simulink model "CF025A_GmFctDiArbn"  (R2013b)
settings: Solver=FixedStepDiscrete  SolverMode=SingleTasking  StartTime=0.0  StopTime=60  FixedStep=0.002  RelTol=1e-3
values from neighbouring files (symbols this model uses):
  GmFctDiArbnEotHwAgThd = DataDict.Calibration    [CF025A_GmFctDiArbn_DataDict.m]
  GmFctDiArbnEotTi = DataDict.Calibration    [CF025A_GmFctDiArbn_DataDict.m]
  GmFctDiArbnOnCentrHwAgThd = DataDict.Calibration    [CF025A_GmFctDiArbn_DataDict.m]
  GmFctDiArbnOnCentrHwTqThd = DataDict.Calibration    [CF025A_GmFctDiArbn_DataDict.m]
  GmFctDiArbnOnCentrTi = DataDict.Calibration    [CF025A_GmFctDiArbn_DataDict.m]
  GmFctDiArbnSrvTi = DataDict.Calibration    [CF025A_GmFctDiArbn_DataDict.m]
  MICROSECTOSEC_ULS_F32 = DataDict.Constant    [CF025A_GmFctDiArbn_DataDict.m]
  ZEROHWAG_HWDEG_F32 = DataDict.Constant    [CF025A_GmFctDiArbn_DataDict.m]
undefined symbols (not defined in the file or in its folder): GmFctDiArbnSts1, LoaSt1
libraries: simulink x7, FixdToFloat x4
(part 1 of 3)
settings Model: Creator=QZWC4R  LastModifiedBy=QZWC4R
settings SolverCC: AutoInsertRateTranBlk=on  InsertRTBMode=Always
settings DataIOCC: LimitDataPoints=off  SaveFormat=Structure  ReturnWorkspaceOutputs=on
settings OptimizationCC: BlockReduction=off  InlineParams=on  ZeroExternalMemoryAtStartup=off  ZeroInternalMemoryAtStartup=off  OptimizeModelRefInitCode=on  LifeSpan=1
settings DebuggingCC: SignalInfNanChecking=error  SignalRangeChecking=warning  UnderspecifiedInitializationDetection=Simplified  SolverPrmCheckMsg=error  InheritedTsInSrcMsg=error  DiscreteInheritContinuousMsg=error  SingleTaskRateTransMsg=error  TasksWithSamePriorityMsg=error  SigSpecEnsureSampleTimeMsg=error  CheckMatrixSingularityMsg=error  ParameterUnderflowMsg=error  ParameterPrecisionLossMsg=error  ParameterTunabilityLossMsg=error  FixptConstUnderflowMsg=warning  FixptConstOverflowMsg=warning  VectorMatrixConversionMsg=error  SignalLabelMismatchMsg=error  UnconnectedInputMsg=error  UnconnectedOutputMsg=error  UnconnectedLineMsg=error  SFcnCompatibilityMsg=error  UniqueDataStoreMsg=warning  BusObjectLabelMismatch=error  RootOutportRequireBusObject=error  AssertControl=DisableAll  ModelReferenceIOMsg=error  ModelReferenceVersionMismatchMessage=warning  ModelReferenceIOMismatchMessage=error  ModelReferenceCSMismatchMessage=warning  ModelReferenceDataLoggingMessage=error  StateNameClashWarn=warning  StrictBusMsg=ErrorOnBusTreatedAsVector  NonBusSignalsTreatedAsBus=error  SFUnexpectedBacktrackingDiag=error  SFInvalidInputDataAccessInChartInitDiag=error  SFNoUnconditionalDefaultTransitionDiag=error  SFTransitionOutsideNaturalParentDiag=error  SFUnconditionalTransitionShadowingDiag=error  SFUndirectedBroadcastEventsDiag=error
settings ModelReferenceCC: ModelReferenceNumInstancesAllowed=Single
settings RTWCC: SystemTargetFile=autosar.tlc  GenCodeOnly=on  TemplateMakefile=ert_default_tmf  Description=AUTOSAR  GenerateReport=on  ProcessScript=autosar_make_rtw_hook  LaunchReport=on
settings CodeAppCC: GenerateComments=off  IgnoreCustomStorageClasses=off  CustomSymbolStrType=$N$R$M  CustomSymbolStrBlkIO=$N$M  SimulinkBlockComments=off
settings STFCustomTargetCC: ParMdlRefBuildCompliant=on  CompOptLevelCompliant=on  IncludeMdlTerminateFcn=off  CombineOutputUpdateFcns=on  SuppressErrorStatus=on  ERTFirstTimeCompliant=on  ERTCustomFileBanners=on  SupportNonFinite=off  SupportComplex=off  SupportContinuousTime=off  SupportNonInlinedSFcns=off  MATLABClassNameForMDSCustomization=Simulink.SoftwareTarget.ERTCustomization  AutosarCompliant=on  GRTInterface=off  SystemTargetFile=autosar.tlc
settings ERTTargetCC: CodeReplacementLibrary=ANSI_C  ConcurrentExecutionCompliant=off  IncludeMdlTerminateFcn=off  SuppressErrorStatus=on  SupportNonFinite=off  SupportComplex=off  ModelStepFunctionPrototypeControlCompliant=off  CPPClassGenCompliant=off  AutosarCompliant=on  InlinedParameterPlacement=NonHierarchical  ERTCustomFileTemplate=example_file_process.tlc  EnableUserReplacementTypes=on

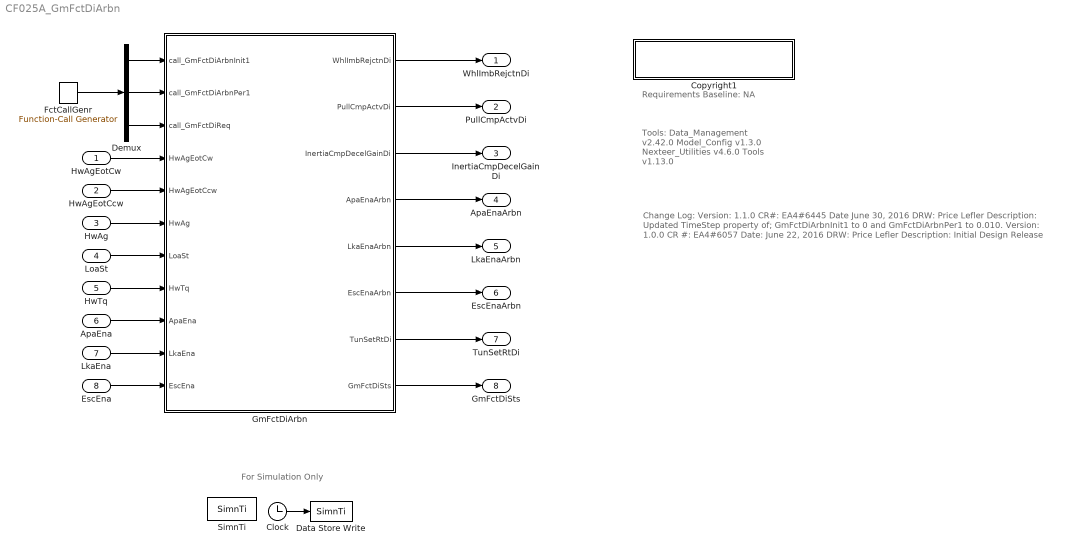
== system CF025A_GmFctDiArbn ==
  note: For Simulation Only
  note: Requirements Baseline:
      | NA
  note: Tools:
      | Data_Management v2.42.0
      | Model_Config v1.3.0
      | Nexteer_Utilities v4.6.0
      | Tools v1.13.0
  note: Change Log:
      |
      | Version: 1.1.0
      | CR#: EA4#6445
      | Date June 30, 2016
      | DRW: Price Lefler
      | Description:
      | 	Updated TimeStep property of; GmFctDiArbnInit1 to 0 and GmFctDiArbnPer1 to 0.010.
      |
      |
      | Version: 1.0.0
      | CR #: EA4#6057
      | Date: June 22, 2016
      | DRW: Price Lefler
      | Description:
      | 	Initial Design Release
  HwAgEotCw : Inport
  HwAgEotCcw : Inport  Port=2
  HwAg : Inport  Port=3
  LoaSt : Inport  Port=4
  HwTq : Inport  Port=5
  ApaEna : Inport  RequirementInfo={'linktype_rmi_doors' '0000bee1 (/E-STEER_New2/Subsytem Spec Documents/Subsystem Core Specs/Customer Functions CF FDR/CF-09 GM Overlay State Handler)' '#42' 'true' '2.1.0-3 GMOSH shall accept an input of an Automated Park Assist 2 Req' '' } %GIDa_2f26ec7d_8ce6_4a1b_a678_32b752ffef3f  Port=6
  LkaEna : Inport  RequirementInfo={'linktype_rmi_doors' '0000bee1 (/E-STEER_New2/Subsytem Spec Documents/Subsystem Core Specs/Customer Functions CF FDR/CF-09 GM Overlay State Handler)' '#48' 'true' '2.1.0-9 GMOSH shall accept an input of a Lane Keeping Assist Request ' '' } %GIDa_32a3aad7_3110_404c_9c6a_95ffa6fb6158  Port=7
  EscEna : Inport  RequirementInfo={'linktype_rmi_doors' '0000bee1 (/E-STEER_New2/Subsytem Spec Documents/Subsystem Core Specs/Customer Functions CF FDR/CF-09 GM Overlay State Handler)' '#51' 'true' '2.1.0-12 GMOSH shall accept an input for a Stability Control Enhanceme' '' } %GIDa_bf71266e_d5fd_41ad_bffd_97b37bc2a8a3  Port=8
  Clock : Clock
  Copyright1 : Subsystem  Description=|  mask(Copyright Information){none=on}
      | Copyright info block.                                               
      |                                                                     
      | Place copyright information at the top of every subsystem in design.
      mask prompts: none "No parameters"
      mask help: Place copyright information at the top of every subsystem in design.
      mask Display:
      | NxtrConf = 'Nexteer Confidential';
      | 
      | sys = bdroot; %handle for the current model ("system")
      | first = get_param(sys,'Created');
      | if(isempty(first))
      |     first = datestr(now,'yyyy');
      | else
      |     first = first(end-3:end);  %year is last four digits
      | end
      | 
      | last = get_param(sys,'LastModifiedDate');
      | if isempty(last)
      |     last = datestr(now,'yyyy');
      | else
      |     last = last(end-3:end);
      | end
      | 
      | if strcmp(first,last)
      |     fprintf('%s\nCopyright  %s Nexteer',NxtrConf,first);
      | else
      |     fprintf('%s\n%s%s-%s Nexteer',NxtrConf,char(169),first,last);
      | end
  Data Store Write : DataStoreWrite  DataStoreName=SimnTi
  Demux : Demux  Outputs=3
  FctCallGenr : simulink/Ports & Subsystems/Function-Call Generator  sample_time=0.010  numberOfIterations=1
  GmFctDiArbn : Subsystem
  SimnTi : DataStoreMemory  DataStoreName=SimnTi
  WhlImbRejctnDi : Outport
  PullCmpActvDi : Outport  Port=2
  InertiaCmpDecelGainDi : Outport  Port=3
  ApaEnaArbn : Outport  Port=4
  LkaEnaArbn : Outport  Port=5
  EscEnaArbn : Outport  Port=6
  TunSetRtDi : Outport  Port=7
  GmFctDiSts : Outport  Port=8
  wires:
  Clock/1 -> Data Store Write/1
  GmFctDiArbn/1(WhlImbRejctnDi) -> WhlImbRejctnDi/1
  GmFctDiArbn/2(PullCmpActvDi) -> PullCmpActvDi/1
  GmFctDiArbn/4(ApaEnaArbn) -> ApaEnaArbn/1
  GmFctDiArbn/5(LkaEnaArbn) -> LkaEnaArbn/1
  GmFctDiArbn/6(EscEnaArbn) -> EscEnaArbn/1
  GmFctDiArbn/7(TunSetRtDi) -> TunSetRtDi/1
  GmFctDiArbn/8(GmFctDiSts) -> GmFctDiSts/1
  HwAgEotCw/1 -> GmFctDiArbn/4(HwAgEotCw)
  HwAgEotCcw/1 -> GmFctDiArbn/5(HwAgEotCcw)
  HwAg/1 -> GmFctDiArbn/6(HwAg)
  LoaSt/1 -> GmFctDiArbn/7(LoaSt)
  HwTq/1 -> GmFctDiArbn/8(HwTq)
  ApaEna/1 -> GmFctDiArbn/9(ApaEna)
  LkaEna/1 -> GmFctDiArbn/10(LkaEna)
  EscEna/1 -> GmFctDiArbn/11(EscEna)
  GmFctDiArbn/3(InertiaCmpDecelGainDi) -> InertiaCmpDecelGainDi/1
  Demux/1 -> GmFctDiArbn/1(call_GmFctDiArbnInit1)
  Demux/2 -> GmFctDiArbn/2(call_GmFctDiArbnPer1)
  Demux/3 -> GmFctDiArbn/3(call_GmFctDiReq)
  FctCallGenr/1 -> Demux/1

== system CF025A_GmFctDiArbn/Copyright1 ==

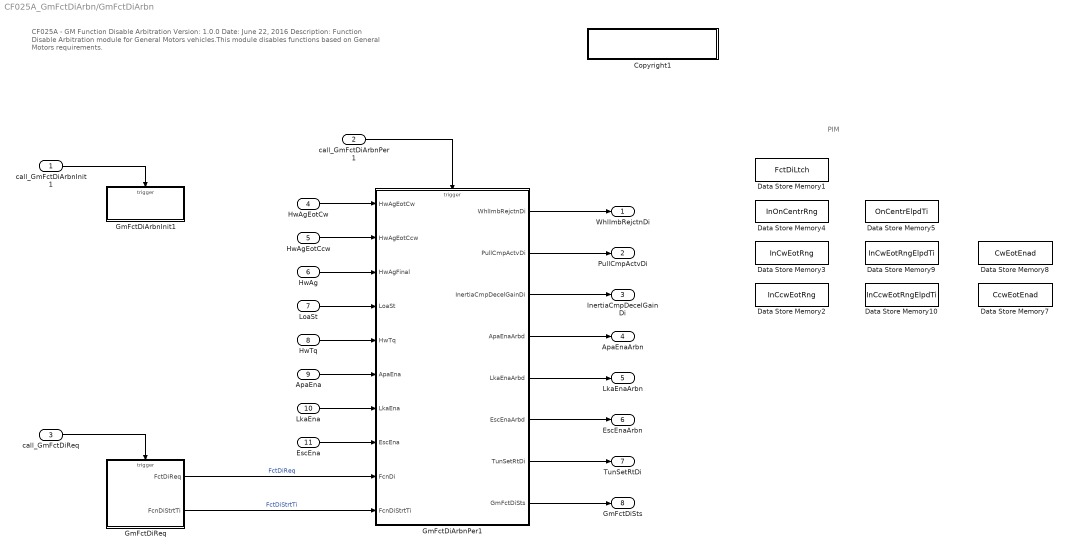
== system CF025A_GmFctDiArbn/GmFctDiArbn ==
  note: CF025A - GM Function Disable Arbitration
      | Version: 1.0.0
      | Date: June 22, 2016
      | Description:
      | 	 Function Disable Arbitration module for General Motors vehicles.This module disables functions based on General Motors requirements.
  note: PIM
  call_GmFctDiArbnInit1 : Inport
  call_GmFctDiArbnPer1 : Inport  Port=2
  call_GmFctDiReq : Inport  Port=3
  HwAgEotCw : Inport  Port=4
  HwAgEotCcw : Inport  Port=5
  HwAg : Inport  Port=6
  LoaSt : Inport  Port=7
  HwTq : Inport  Port=8
  ApaEna : Inport  RequirementInfo={'linktype_rmi_doors' '0000bee1 (/E-STEER_New2/Subsytem Spec Documents/Subsystem Core Specs/Customer Functions CF FDR/CF-09 GM Overlay State Handler)' '#42' 'true' '2.1.0-3 GMOSH shall accept an input of an Automated Park Assist 2 Req' '' } %GIDa_2c17c048_e723_4115_94ae_0e322b12958e  Port=9
  LkaEna : Inport  RequirementInfo={'linktype_rmi_doors' '0000bee1 (/E-STEER_New2/Subsytem Spec Documents/Subsystem Core Specs/Customer Functions CF FDR/CF-09 GM Overlay State Handler)' '#48' 'true' '2.1.0-9 GMOSH shall accept an input of a Lane Keeping Assist Request ' '' } %GIDa_a26b014d_6879_4602_9502_03f06376d044  Port=10
  EscEna : Inport  RequirementInfo={'linktype_rmi_doors' '0000bee1 (/E-STEER_New2/Subsytem Spec Documents/Subsystem Core Specs/Customer Functions CF FDR/CF-09 GM Overlay State Handler)' '#51' 'true' '2.1.0-12 GMOSH shall accept an input for a Stability Control Enhanceme' '' } %GIDa_8379b319_8fa0_4ff7_8623_9b680c80b153  Port=11
  Copyright1 : Subsystem  Description=|  mask(Copyright Information){none=on}
      | Copyright info block.                                               
      |                                                                     
      | Place copyright information at the top of every subsystem in design.
      mask prompts: none "No parameters"
      mask help: Place copyright information at the top of every subsystem in design.
      mask Display:
      | NxtrConf = 'Nexteer Confidential';
      | 
      | sys = bdroot; %handle for the current model ("system")
      | first = get_param(sys,'Created');
      | if(isempty(first))
      |     first = datestr(now,'yyyy');
      | else
      |     first = first(end-3:end);  %year is last four digits
      | end
      | 
      | last = get_param(sys,'LastModifiedDate');
      | if isempty(last)
      |     last = datestr(now,'yyyy');
      | else
      |     last = last(end-3:end);
      | end
      | 
      | if strcmp(first,last)
      |     fprintf('%s\nCopyright  %s Nexteer',NxtrConf,first);
      | else
      |     fprintf('%s\n%s%s-%s Nexteer',NxtrConf,char(169),first,last);
      | end
  Data Store Memory1 : DataStoreMemory  DataStoreName=FctDiLtch  StateMustResolveToSignalObject=on
  Data Store Memory10 : DataStoreMemory  DataStoreName=InCcwEotRngElpdTi  StateMustResolveToSignalObject=on
  Data Store Memory2 : DataStoreMemory  DataStoreName=InCcwEotRng  StateMustResolveToSignalObject=on
  Data Store Memory3 : DataStoreMemory  DataStoreName=InCwEotRng  StateMustResolveToSignalObject=on
  Data Store Memory4 : DataStoreMemory  DataStoreName=InOnCentrRng  StateMustResolveToSignalObject=on
  Data Store Memory5 : DataStoreMemory  DataStoreName=OnCentrElpdTi  StateMustResolveToSignalObject=on
  Data Store Memory7 : DataStoreMemory  DataStoreName=CcwEotEnad  StateMustResolveToSignalObject=on
  Data Store Memory8 : DataStoreMemory  DataStoreName=CwEotEnad  StateMustResolveToSignalObject=on
  Data Store Memory9 : DataStoreMemory  DataStoreName=InCwEotRngElpdTi  StateMustResolveToSignalObject=on
  GmFctDiArbnInit1 : Subsystem  TreatAsAtomicUnit=on
  GmFctDiArbnPer1 : Subsystem  TreatAsAtomicUnit=on
  GmFctDiReq : Subsystem  TreatAsAtomicUnit=on
  WhlImbRejctnDi : Outport
  PullCmpActvDi : Outport  Port=2
  InertiaCmpDecelGainDi : Outport  Port=3
  ApaEnaArbn : Outport  Port=4
  LkaEnaArbn : Outport  Port=5
  EscEnaArbn : Outport  Port=6
  TunSetRtDi : Outport  Port=7
  GmFctDiSts : Outport  Port=8
  wires:
  call_GmFctDiArbnInit1/1 -> GmFctDiArbnInit1/Trigger
  call_GmFctDiArbnPer1/1 -> GmFctDiArbnPer1/Trigger
  HwTq/1 -> GmFctDiArbnPer1/5(HwTq)
  LoaSt/1 -> GmFctDiArbnPer1/4(LoaSt)
  HwAg/1 -> GmFctDiArbnPer1/3(HwAgFinal)
  HwAgEotCcw/1 -> GmFctDiArbnPer1/2(HwAgEotCcw)
  HwAgEotCw/1 -> GmFctDiArbnPer1/1(HwAgEotCw)
  GmFctDiArbnPer1/1(WhlImbRejctnDi) -> WhlImbRejctnDi/1
  GmFctDiArbnPer1/2(PullCmpActvDi) -> PullCmpActvDi/1
  GmFctDiArbnPer1/3(InertiaCmpDecelGainDi) -> InertiaCmpDecelGainDi/1
  GmFctDiArbnPer1/4(ApaEnaArbd) -> ApaEnaArbn/1
  GmFctDiArbnPer1/5(LkaEnaArbd) -> LkaEnaArbn/1
  GmFctDiArbnPer1/6(EscEnaArbd) -> EscEnaArbn/1
  call_GmFctDiReq/1 -> GmFctDiReq/Trigger
  GmFctDiReq/1(FctDiReq) -> GmFctDiArbnPer1/9(FcnDi)  "FctDiReq"
  ApaEna/1 -> GmFctDiArbnPer1/6(ApaEna)
  LkaEna/1 -> GmFctDiArbnPer1/7(LkaEna)
  EscEna/1 -> GmFctDiArbnPer1/8(EscEna)
  GmFctDiArbnPer1/7(TunSetRtDi) -> TunSetRtDi/1
  GmFctDiArbnPer1/8(GmFctDiSts) -> GmFctDiSts/1
  GmFctDiReq/2(FcnDiStrtTi) -> GmFctDiArbnPer1/10(FcnDiStrtTi)  "FctDiStrtTi"

== system CF025A_GmFctDiArbn/GmFctDiArbn/Copyright1 ==

== system CF025A_GmFctDiArbn/GmFctDiArbn/GmFctDiArbnInit1 ==
  function : TriggerPort  TriggerType=function-call
  Copyright1 : Subsystem  Description=|  mask(Copyright Information){none=on}
      | Copyright info block.                                               
      |                                                                     
      | Place copyright information at the top of every subsystem in design.
      mask prompts: none "No parameters"
      mask help: Place copyright information at the top of every subsystem in design.
      mask Display:
      | NxtrConf = 'Nexteer Confidential';
      | 
      | sys = bdroot; %handle for the current model ("system")
      | first = get_param(sys,'Created');
      | if(isempty(first))
      |     first = datestr(now,'yyyy');
      | else
      |     first = first(end-3:end);  %year is last four digits
      | end
      | 
      | last = get_param(sys,'LastModifiedDate');
      | if isempty(last)
      |     last = datestr(now,'yyyy');
      | else
      |     last = last(end-3:end);
      | end
      | 
      | if strcmp(first,last)
      |     fprintf('%s\nCopyright  %s Nexteer',NxtrConf,first);
      | else
      |     fprintf('%s\n%s%s-%s Nexteer',NxtrConf,char(169),first,last);
      | end

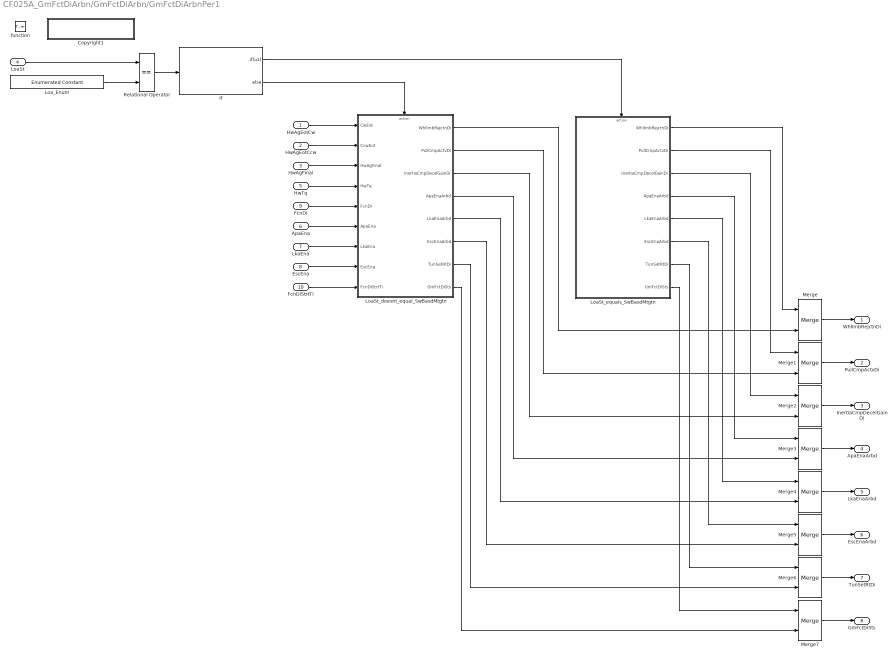
== system CF025A_GmFctDiArbn/GmFctDiArbn/GmFctDiArbnPer1 ==
  HwAgEotCw : Inport
  HwAgEotCcw : Inport  Port=2
  HwAgFinal : Inport  Port=3
  LoaSt : Inport  Port=4
  HwTq : Inport  Port=5
  ApaEna : Inport  RequirementInfo={'linktype_rmi_doors' '0000bee1 (/E-STEER_New2/Subsytem Spec Documents/Subsystem Core Specs/Customer Functions CF FDR/CF-09 GM Overlay State Handler)' '#42' 'true' '2.1.0-3 GMOSH shall accept an input of an Automated Park Assist 2 Req' '' } %GIDa_eb388981_6ca0_4296_8e81_aef3a122a5ab  Port=6
  LkaEna : Inport  RequirementInfo={'linktype_rmi_doors' '0000bee1 (/E-STEER_New2/Subsytem Spec Documents/Subsystem Core Specs/Customer Functions CF FDR/CF-09 GM Overlay State Handler)' '#48' 'true' '2.1.0-9 GMOSH shall accept an input of a Lane Keeping Assist Request ' '' } %GIDa_cd443268_1945_4186_bec6_c8c383fdf52f  Port=7
  EscEna : Inport  RequirementInfo={'linktype_rmi_doors' '0000bee1 (/E-STEER_New2/Subsytem Spec Documents/Subsystem Core Specs/Customer Functions CF FDR/CF-09 GM Overlay State Handler)' '#51' 'true' '2.1.0-12 GMOSH shall accept an input for a Stability Control Enhanceme' '' } %GIDa_e4a9320c_e488_484d_a205_861b0d5f4219  Port=8
  FcnDi : Inport  Port=9
  FcnDiStrtTi : Inport  Port=10  OutDataTypeStr=uint32
  function : TriggerPort  TriggerType=function-call
  Copyright1 : Subsystem  Description=|  mask(Copyright Information){none=on}
      | Copyright info block.                                               
      |                                                                     
      | Place copyright information at the top of every subsystem in design.
      mask prompts: none "No parameters"
      mask help: Place copyright information at the top of every subsystem in design.
      mask Display:
      | NxtrConf = 'Nexteer Confidential';
      | 
      | sys = bdroot; %handle for the current model ("system")
      | first = get_param(sys,'Created');
      | if(isempty(first))
      |     first = datestr(now,'yyyy');
      | else
      |     first = first(end-3:end);  %year is last four digits
      | end
      | 
      | last = get_param(sys,'LastModifiedDate');
      | if isempty(last)
      |     last = datestr(now,'yyyy');
      | else
      |     last = last(end-3:end);
      | end
      | 
      | if strcmp(first,last)
      |     fprintf('%s\nCopyright  %s Nexteer',NxtrConf,first);
      | else
      |     fprintf('%s\n%s%s-%s Nexteer',NxtrConf,char(169),first,last);
      | end
  If : If  IfExpression=u1
  LoaSt_doesnt_equal_SwBasdMtgtn : Subsystem  TreatAsAtomicUnit=on
  LoaSt_equals_SwBasdMtgtn : Subsystem  TreatAsAtomicUnit=on
  Loa_Enum : simulink/Sources/Enumerated Constant  OutDataTypeStr=Enum: LoaSt1  Value=LoaSt1.LOAST_SWBASDMTGTN  SampleTime=inf
  Merge{,1..7} (8 alike) : Merge
  Relational Operator : RelationalOperator  Operator===  OutDataTypeStr=boolean
  WhlImbRejctnDi : Outport
  PullCmpActvDi : Outport  Port=2
  InertiaCmpDecelGainDi : Outport  Port=3
  ApaEnaArbd : Outport  Port=4
  LkaEnaArbd : Outport  Port=5
  EscEnaArbd : Outport  Port=6
  TunSetRtDi : Outport  Port=7
  GmFctDiSts : Outport  Port=8
  wires:
  LoaSt/1 -> Relational Operator/1
  Loa_Enum/1 -> Relational Operator/2
  If/1 -> LoaSt_equals_SwBasdMtgtn/Action
  Merge/1 -> WhlImbRejctnDi/1
  Merge1/1 -> PullCmpActvDi/1
  Merge2/1 -> InertiaCmpDecelGainDi/1
  Merge3/1 -> ApaEnaArbd/1
  Merge4/1 -> LkaEnaArbd/1
  Merge5/1 -> EscEnaArbd/1
  If/2 -> LoaSt_doesnt_equal_SwBasdMtgtn/Action
  HwAgEotCw/1 -> LoaSt_doesnt_equal_SwBasdMtgtn/1(CwEot)
  HwAgEotCcw/1 -> LoaSt_doesnt_equal_SwBasdMtgtn/2(CcwEot)
  HwAgFinal/1 -> LoaSt_doesnt_equal_SwBasdMtgtn/3(HwAgFinal)
  HwTq/1 -> LoaSt_doesnt_equal_SwBasdMtgtn/4(HwTq)
  FcnDi/1 -> LoaSt_doesnt_equal_SwBasdMtgtn/5(FcnDi)
  ApaEna/1 -> LoaSt_doesnt_equal_SwBasdMtgtn/6(ApaEna)
  LkaEna/1 -> LoaSt_doesnt_equal_SwBasdMtgtn/7(LkaEna)
  EscEna/1 -> LoaSt_doesnt_equal_SwBasdMtgtn/8(EscEna)
  Merge6/1 -> TunSetRtDi/1
  Merge7/1 -> GmFctDiSts/1
  Relational Operator/1 -> If/1
  LoaSt_equals_SwBasdMtgtn/1(WhlImbRejctnDi) -> Merge/1
  LoaSt_doesnt_equal_SwBasdMtgtn/1(WhlImbRejctnDi) -> Merge/2
  LoaSt_equals_SwBasdMtgtn/2(PullCmpActvDi) -> Merge1/1
  LoaSt_doesnt_equal_SwBasdMtgtn/2(PullCmpActvDi) -> Merge1/2
  LoaSt_equals_SwBasdMtgtn/3(InertiaCmpDecelGainDi) -> Merge2/1
  LoaSt_doesnt_equal_SwBasdMtgtn/3(InertiaCmpDecelGainDi) -> Merge2/2
  LoaSt_equals_SwBasdMtgtn/4(ApaEnaArbd) -> Merge3/1
  LoaSt_doesnt_equal_SwBasdMtgtn/4(ApaEnaArbd) -> Merge3/2
  LoaSt_equals_SwBasdMtgtn/5(LkaEnaArbd) -> Merge4/1
  LoaSt_doesnt_equal_SwBasdMtgtn/5(LkaEnaArbd) -> Merge4/2
  LoaSt_equals_SwBasdMtgtn/6(EscEnaArbd) -> Merge5/1
  LoaSt_equals_SwBasdMtgtn/7(TunSetRtDi) -> Merge6/1
  LoaSt_doesnt_equal_SwBasdMtgtn/7(TunSetRtDi) -> Merge6/2
  LoaSt_doesnt_equal_SwBasdMtgtn/6(EscEnaArbd) -> Merge5/2
  LoaSt_equals_SwBasdMtgtn/8(GmFctDiSts) -> Merge7/1
  LoaSt_doesnt_equal_SwBasdMtgtn/8(GmFctDiSts) -> Merge7/2
  FcnDiStrtTi/1 -> LoaSt_doesnt_equal_SwBasdMtgtn/9(FcnDiStrtTi)

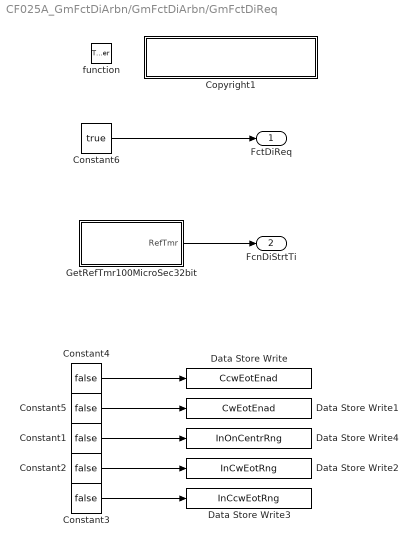
== system CF025A_GmFctDiArbn/GmFctDiArbn/GmFctDiReq ==
  function : TriggerPort  TriggerType=function-call
  Constant{1..5} (5 alike) : Constant  Value=false
  Constant6 : Constant  Value=true
  Copyright1 : Subsystem  Description=|  mask(Copyright Information){none=on}
      | Copyright info block.                                               
      |                                                                     
      | Place copyright information at the top of every subsystem in design.
      mask prompts: none "No parameters"
      mask help: Place copyright information at the top of every subsystem in design.
      mask Display:
      | NxtrConf = 'Nexteer Confidential';
      | 
      | sys = bdroot; %handle for the current model ("system")
      | first = get_param(sys,'Created');
      | if(isempty(first))
      |     first = datestr(now,'yyyy');
      | else
      |     first = first(end-3:end);  %year is last four digits
      | end
      | 
      | last = get_param(sys,'LastModifiedDate');
      | if isempty(last)
      |     last = datestr(now,'yyyy');
      | else
      |     last = last(end-3:end);
      | end
      | 
      | if strcmp(first,last)
      |     fprintf('%s\nCopyright  %s Nexteer',NxtrConf,first);
      | else
      |     fprintf('%s\n%s%s-%s Nexteer',NxtrConf,char(169),first,last);
      | end
  Data Store Write : DataStoreWrite  DataStoreName=CcwEotEnad
  Data Store Write1 : DataStoreWrite  DataStoreName=CwEotEnad
  Data Store Write2 : DataStoreWrite  DataStoreName=InCwEotRng
  Data Store Write3 : DataStoreWrite  DataStoreName=InCcwEotRng
  Data Store Write4 : DataStoreWrite  DataStoreName=InOnCentrRng
  GetRefTmr100MicroSec32bit : Subsystem
  FctDiReq : Outport  InitialOutput=false
      settings: AttributesFormatString=|
      | Output IC: %<InitialOutput>
      | For Simulation Only.
  FcnDiStrtTi : Outport  Port=2
  wires:
  GetRefTmr100MicroSec32bit/1(RefTmr) -> FcnDiStrtTi/1
  Constant4/1 -> Data Store Write/1
  Constant5/1 -> Data Store Write1/1
  Constant1/1 -> Data Store Write4/1
  Constant2/1 -> Data Store Write2/1
  Constant3/1 -> Data Store Write3/1
  Constant6/1 -> FctDiReq/1

== system CF025A_GmFctDiArbn/GmFctDiArbn/GmFctDiArbnInit1/Copyright1 ==

== system CF025A_GmFctDiArbn/GmFctDiArbn/GmFctDiArbnPer1/Copyright1 ==

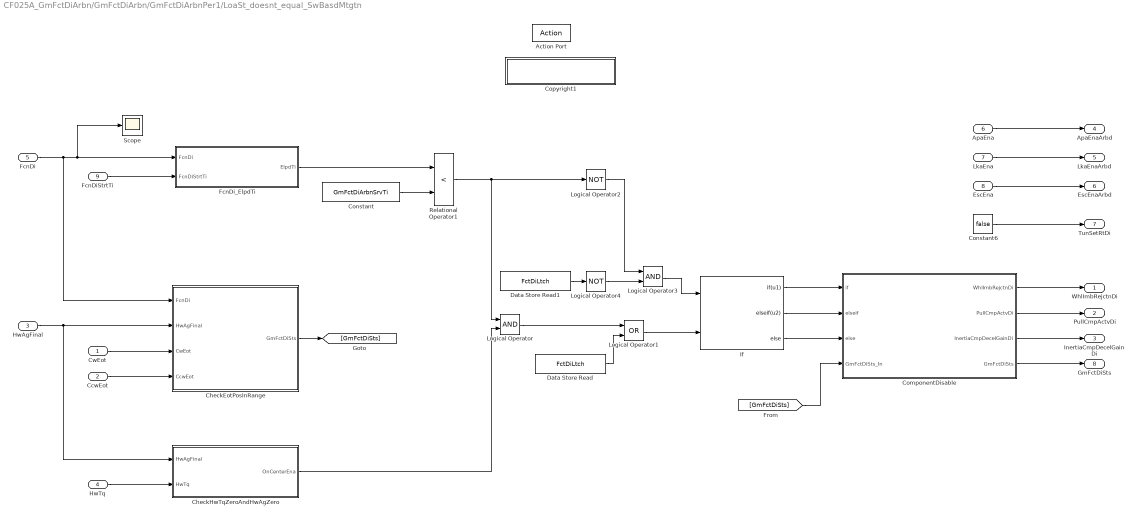
== system CF025A_GmFctDiArbn/GmFctDiArbn/GmFctDiArbnPer1/LoaSt_doesnt_equal_SwBasdMtgtn ==
  CwEot : Inport
  CcwEot : Inport  Port=2
  HwAgFinal : Inport  Port=3
  HwTq : Inport  Port=4
  FcnDi : Inport  Port=5
  ApaEna : Inport  RequirementInfo={'linktype_rmi_doors' '0000bee1 (/E-STEER_New2/Subsytem Spec Documents/Subsystem Core Specs/Customer Functions CF FDR/CF-09 GM Overlay State Handler)' '#42' 'true' '2.1.0-3 GMOSH shall accept an input of an Automated Park Assist 2 Req' '' } %GIDa_4c3b4a4d_4bd1_4ac6_b43d_6a3658ff9675  Port=6
  LkaEna : Inport  RequirementInfo={'linktype_rmi_doors' '0000bee1 (/E-STEER_New2/Subsytem Spec Documents/Subsystem Core Specs/Customer Functions CF FDR/CF-09 GM Overlay State Handler)' '#48' 'true' '2.1.0-9 GMOSH shall accept an input of a Lane Keeping Assist Request ' '' } %GIDa_aabf4122_7ea8_4387_9a0b_41aa0f5fdb39  Port=7
  EscEna : Inport  RequirementInfo={'linktype_rmi_doors' '0000bee1 (/E-STEER_New2/Subsytem Spec Documents/Subsystem Core Specs/Customer Functions CF FDR/CF-09 GM Overlay State Handler)' '#51' 'true' '2.1.0-12 GMOSH shall accept an input for a Stability Control Enhanceme' '' } %GIDa_db93f32a_9bac_4ded_8002_6031963bead0  Port=8
  FcnDiStrtTi : Inport  Port=9  OutDataTypeStr=uint32
  Action Port : ActionPort  ActionType=else
  CheckEotPosInRange : Subsystem
  CheckHwTqZeroAndHwAgZero : Subsystem
  ComponentDisable : Subsystem
  Constant : Constant  Value=GmFctDiArbnSrvTi
  Constant6 : Constant  Value=false  OutDataTypeStr=boolean
  Copyright1 : Subsystem  Description=|  mask(Copyright Information){none=on}
      | Copyright info block.                                               
      |                                                                     
      | Place copyright information at the top of every subsystem in design.
      mask prompts: none "No parameters"
      mask help: Place copyright information at the top of every subsystem in design.
      mask Display:
      | NxtrConf = 'Nexteer Confidential';
      | 
      | sys = bdroot; %handle for the current model ("system")
      | first = get_param(sys,'Created');
      | if(isempty(first))
      |     first = datestr(now,'yyyy');
      | else
      |     first = first(end-3:end);  %year is last four digits
      | end
      | 
      | last = get_param(sys,'LastModifiedDate');
      | if isempty(last)
      |     last = datestr(now,'yyyy');
      | else
      |     last = last(end-3:end);
      | end
      | 
      | if strcmp(first,last)
      |     fprintf('%s\nCopyright  %s Nexteer',NxtrConf,first);
      | else
      |     fprintf('%s\n%s%s-%s Nexteer',NxtrConf,char(169),first,last);
      | end
  Data Store Read : DataStoreRead  DataStoreName=FctDiLtch
  Data Store Read1 : DataStoreRead  DataStoreName=FctDiLtch
  FcnDi_ElpdTi : Subsystem
  If : If  NumInputs=2  IfExpression=u1  ElseIfExpressions=u2
  Logical Operator : Logic  AllPortsSameDT=off  OutDataTypeStr=boolean
  Logical Operator1 : Logic  Operator=OR  AllPortsSameDT=off  OutDataTypeStr=boolean
  Logical Operator2 : Logic  Operator=NOT  AllPortsSameDT=off  OutDataTypeStr=boolean
  Logical Operator3 : Logic  AllPortsSameDT=off  OutDataTypeStr=boolean
  Logical Operator4 : Logic  Operator=NOT  AllPortsSameDT=off  OutDataTypeStr=boolean
  Relational Operator1 : RelationalOperator  Operator=<  OutDataTypeStr=boolean
  Scope : Scope
      settings: SaveName=ScopeData5
  WhlImbRejctnDi : Outport
  PullCmpActvDi : Outport  Port=2
  InertiaCmpDecelGainDi : Outport  Port=3
  ApaEnaArbd : Outport  Port=4
  LkaEnaArbd : Outport  Port=5
  EscEnaArbd : Outport  Port=6
  TunSetRtDi : Outport  Port=7
  GmFctDiSts : Outport  Port=8
  wires:
  FcnDi_ElpdTi/1(ElpdTi) -> Relational Operator1/1
  CwEot/1 -> CheckEotPosInRange/3(CwEot)
  CcwEot/1 -> CheckEotPosInRange/4(CcwEot)
  HwAgFinal/1 -> CheckHwTqZeroAndHwAgZero/1(HwAgFinal), CheckEotPosInRange/2(HwAgFinal)
  HwTq/1 -> CheckHwTqZeroAndHwAgZero/2(HwTq)
  CheckHwTqZeroAndHwAgZero/1(OnCenterEna) -> Logical Operator/2
  Constant/1 -> Relational Operator1/2
  Relational Operator1/1 -> Logical Operator2/1, Logical Operator/1
  Logical Operator/1 -> Logical Operator1/1
  Logical Operator1/1 -> If/2
  Data Store Read/1 -> Logical Operator1/2
  ApaEna/1 -> ApaEnaArbd/1
  LkaEna/1 -> LkaEnaArbd/1
  EscEna/1 -> EscEnaArbd/1
  Constant6/1 -> TunSetRtDi/1
  If/1 -> ComponentDisable/1(if)
  If/2 -> ComponentDisable/2(elseif)
  If/3 -> ComponentDisable/3(else)
  ComponentDisable/1(WhlImbRejctnDi) -> WhlImbRejctnDi/1
  ComponentDisable/2(PullCmpActvDi) -> PullCmpActvDi/1
  ComponentDisable/3(InertiaCmpDecelGainDi) -> InertiaCmpDecelGainDi/1
  ComponentDisable/4(GmFctDiSts) -> GmFctDiSts/1
  CheckEotPosInRange/1(GmFctDiSts) -> [GmFctDiSts]
  [GmFctDiSts] -> ComponentDisable/4(GmFctDiSts_In)
  FcnDiStrtTi/1 -> FcnDi_ElpdTi/2(FcnDiStrtTi)
  Data Store Read1/1 -> Logical Operator4/1
  Logical Operator4/1 -> Logical Operator3/2
  FcnDi/1 -> Scope/1, FcnDi_ElpdTi/1(FcnDi), CheckEotPosInRange/1(FcnDi)
  Logical Operator2/1 -> Logical Operator3/1
  Logical Operator3/1 -> If/1

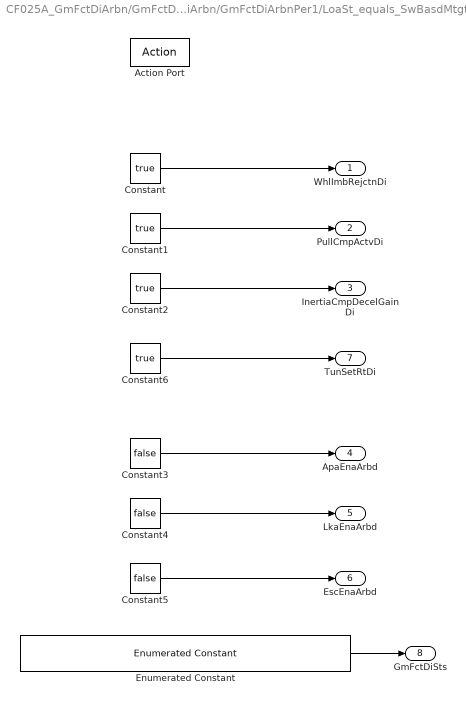
== system CF025A_GmFctDiArbn/GmFctDiArbn/GmFctDiArbnPer1/LoaSt_equals_SwBasdMtgtn ==
  Action Port : ActionPort  ActionType=then
  Constant{,1..2,6} (4 alike) : Constant  Value=true  OutDataTypeStr=boolean
  Constant3 : Constant  Value=false  OutDataTypeStr=boolean
  Constant4 : Constant  Value=false  OutDataTypeStr=boolean
  Constant5 : Constant  Value=false  OutDataTypeStr=boolean
  Enumerated Constant : simulink/Sources/Enumerated Constant  OutDataTypeStr=Enum: GmFctDiArbnSts1  Value=GmFctDiArbnSts1.GMFCTDIARBNSTS_SWBASDMTGTNFAIL  SampleTime=inf
  WhlImbRejctnDi : Outport
  PullCmpActvDi : Outport  Port=2
  InertiaCmpDecelGainDi : Outport  Port=3
  ApaEnaArbd : Outport  Port=4
  LkaEnaArbd : Outport  Port=5
  EscEnaArbd : Outport  Port=6
  TunSetRtDi : Outport  Port=7
  GmFctDiSts : Outport  Port=8
  wires:
  Constant/1 -> WhlImbRejctnDi/1
  Constant1/1 -> PullCmpActvDi/1
  Constant2/1 -> InertiaCmpDecelGainDi/1
  Constant3/1 -> ApaEnaArbd/1
  Constant4/1 -> LkaEnaArbd/1
  Constant5/1 -> EscEnaArbd/1
  Constant6/1 -> TunSetRtDi/1
  Enumerated Constant/1 -> GmFctDiSts/1

== system CF025A_GmFctDiArbn/GmFctDiArbn/GmFctDiReq/Copyright1 ==

== system CF025A_GmFctDiArbn/GmFctDiArbn/GmFctDiReq/GetRefTmr100MicroSec32bit ==
  note: 1 count = 100 uSec
  note: seconds
  note: microseconds
  note: counts
  note: Wrap-to-zero
  note: GetRefTmr100MicroSec32bit
  note: Created Aug 18, 2015
      | Modified Oct 21, 2015
      | Modified Oct 30, 2015
      | Kevin Derry
  CopyRight2 : Subsystem  Description=|  mask(Copyright Information){none=on}
      | Copyright info block.                                               
      |                                                                     
      | Place copyright information at the top of every subsystem in design.
      mask prompts: none "No parameters"
      mask help: Place copyright information at the top of every subsystem in design.
      mask Display:
      | NxtrConf = 'Nexteer Confidential';
      | 
      | sys = bdroot; %handle for the current model ("system")
      | first = get_param(sys,'Created');
      | if(isempty(first))
      |     first = datestr(now,'yyyy');
      | else
      |     first = first(end-3:end);  %year is last four digits
      | end
      | 
      | last = get_param(sys,'LastModifiedDate');
      | if isempty(last)
      |     last = datestr(now,'yyyy');
      | else
      |     last = last(end-3:end);
      | end
      | 
      | if strcmp(first,last)
      |     fprintf('%s -- Copyright %s Nexteer',NxtrConf,first)
      | else
      |     fprintf('%s -- %s%s- %s Nexteer',NxtrConf,char(169),first,last)
      | end
  Count per uSec : Constant  Value=0.01
  Data Store Read1 : DataStoreRead  DataStoreName=SimnTi
  Data Type Conversion1 : DataTypeConversion  OutDataTypeStr=uint32
  Divide1 : Product  Inputs=**
  Divide2 : Product  Inputs=*/
  Max Counts : Constant  Value=2^32-1
  Product1 : Product
  Product2 : Product
  Rounding : Rounding
  Subtract1 : Sum  Inputs=+-
  uSec per Sec : Constant  Value=1000000
  RefTmr : Outport
  wires:
  Product2/1 -> Subtract1/2
  Subtract1/1 -> Data Type Conversion1/1
  Rounding/1 -> Product2/1
  Divide2/1 -> Rounding/1
  Max Counts/1 -> Divide2/2, Product2/2
  Divide1/1 -> Divide2/1, Subtract1/1
  Product1/1 -> Divide1/1
  Count per uSec/1 -> Divide1/2
  uSec per Sec/1 -> Product1/2
  Data Type Conversion1/1 -> RefTmr/1
  Data Store Read1/1 -> Product1/1

== system CF025A_GmFctDiArbn/GmFctDiArbn/GmFctDiArbnPer1/LoaSt_doesnt_equal_SwBasdMtgtn/CheckEotPosInRange ==
  FcnDi : Inport
  HwAgFinal : Inport  Port=2
  CwEot : Inport  Port=3
  CcwEot : Inport  Port=4
  Copyright1 : Subsystem  Description=|  mask(Copyright Information){none=on}
      | Copyright info block.                                               
      |                                                                     
      | Place copyright information at the top of every subsystem in design.
      mask prompts: none "No parameters"
      mask help: Place copyright information at the top of every subsystem in design.
      mask Display:
      | NxtrConf = 'Nexteer Confidential';
      | 
      | sys = bdroot; %handle for the current model ("system")
      | first = get_param(sys,'Created');
      | if(isempty(first))
      |     first = datestr(now,'yyyy');
      | else
      |     first = first(end-3:end);  %year is last four digits
      | end
      | 
      | last = get_param(sys,'LastModifiedDate');
      | if isempty(last)
      |     last = datestr(now,'yyyy');
      | else
      |     last = last(end-3:end);
      | end
      | 
      | if strcmp(first,last)
      |     fprintf('%s\nCopyright  %s Nexteer',NxtrConf,first);
      | else
      |     fprintf('%s\n%s%s-%s Nexteer',NxtrConf,char(169),first,last);
      | end
  If : If  IfExpression=u1
  InProc : Subsystem  TreatAsAtomicUnit=on
  Merge : Merge
  Wait : Subsystem  TreatAsAtomicUnit=on
  GmFctDiSts : Outport
  wires:
  HwAgFinal/1 -> InProc/1(HwAgFinal)
  FcnDi/1 -> If/1
  CwEot/1 -> InProc/2(CwEot)
  If/2 -> Wait/Action
  CcwEot/1 -> InProc/3(CcwEot)
  If/1 -> InProc/Action
  InProc/1(GmFctDiSts_InProc) -> Merge/1
  Wait/1(GmFctDiSts_Wait) -> Merge/2
  Merge/1 -> GmFctDiSts/1

== system CF025A_GmFctDiArbn/GmFctDiArbn/GmFctDiArbnPer1/LoaSt_doesnt_equal_SwBasdMtgtn/CheckHwTqZeroAndHwAgZero ==
  HwAgFinal : Inport
  HwTq : Inport  Port=2
  Copyright1 : Subsystem  Description=|  mask(Copyright Information){none=on}
      | Copyright info block.                                               
      |                                                                     
      | Place copyright information at the top of every subsystem in design.
      mask prompts: none "No parameters"
      mask help: Place copyright information at the top of every subsystem in design.
      mask Display:
      | NxtrConf = 'Nexteer Confidential';
      | 
      | sys = bdroot; %handle for the current model ("system")
      | first = get_param(sys,'Created');
      | if(isempty(first))
      |     first = datestr(now,'yyyy');
      | else
      |     first = first(end-3:end);  %year is last four digits
      | end
      | 
      | last = get_param(sys,'LastModifiedDate');
      | if isempty(last)
      |     last = datestr(now,'yyyy');
      | else
      |     last = last(end-3:end);
      | end
      | 
      | if strcmp(first,last)
      |     fprintf('%s\nCopyright  %s Nexteer',NxtrConf,first);
      | else
      |     fprintf('%s\n%s%s-%s Nexteer',NxtrConf,char(169),first,last);
      | end
  Data Store Read : DataStoreRead  DataStoreName=CwEotEnad
  Data Store Read1 : DataStoreRead  DataStoreName=CcwEotEnad
  If : If  IfExpression=u1  ShowElse=off
  IfBothEotElpdTimeMet : Subsystem  TreatAsAtomicUnit=on
  Logical Operator1 : Logic  AllPortsSameDT=off  OutDataTypeStr=boolean
  OnCenterEna : Outport
  wires:
  Data Store Read1/1 -> Logical Operator1/1
  Data Store Read/1 -> Logical Operator1/2
  Logical Operator1/1 -> If/1
  If/1 -> IfBothEotElpdTimeMet/Action
  HwAgFinal/1 -> IfBothEotElpdTimeMet/1(HwAgFinal)
  HwTq/1 -> IfBothEotElpdTimeMet/2(HwTq)
  IfBothEotElpdTimeMet/1(OnCenterEna) -> OnCenterEna/1

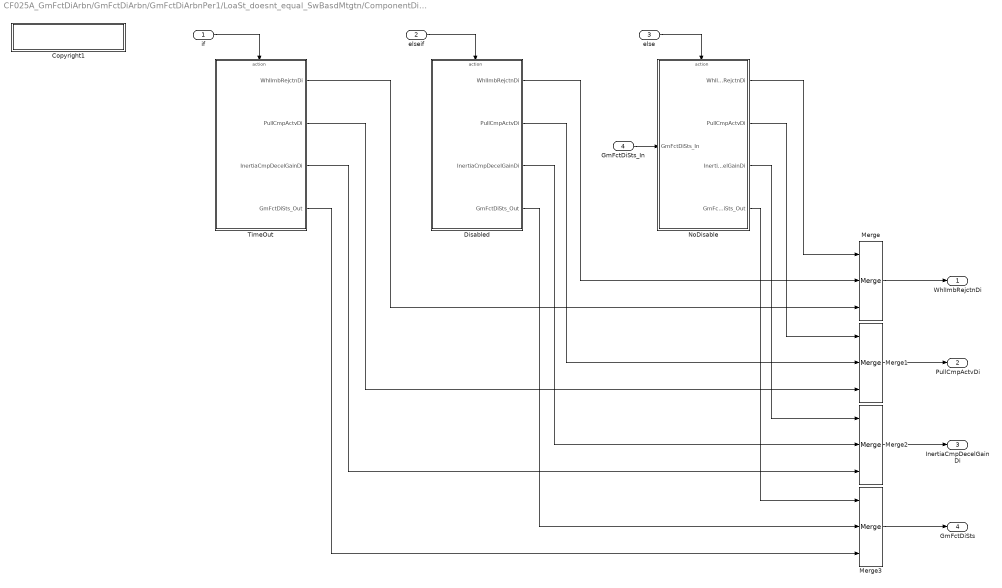
== system CF025A_GmFctDiArbn/GmFctDiArbn/GmFctDiArbnPer1/LoaSt_doesnt_equal_SwBasdMtgtn/ComponentDisable ==
  if : Inport
  elseif : Inport  Port=2
  else : Inport  Port=3
  GmFctDiSts_In : Inport  Port=4
  Copyright1 : Subsystem  Description=|  mask(Copyright Information){none=on}
      | Copyright info block.                                               
      |                                                                     
      | Place copyright information at the top of every subsystem in design.
      mask prompts: none "No parameters"
      mask help: Place copyright information at the top of every subsystem in design.
      mask Display:
      | NxtrConf = 'Nexteer Confidential';
      | 
      | sys = bdroot; %handle for the current model ("system")
      | first = get_param(sys,'Created');
      | if(isempty(first))
      |     first = datestr(now,'yyyy');
      | else
      |     first = first(end-3:end);  %year is last four digits
      | end
      | 
      | last = get_param(sys,'LastModifiedDate');
      | if isempty(last)
      |     last = datestr(now,'yyyy');
      | else
      |     last = last(end-3:end);
      | end
      | 
      | if strcmp(first,last)
      |     fprintf('%s\nCopyright  %s Nexteer',NxtrConf,first);
      | else
      |     fprintf('%s\n%s%s-%s Nexteer',NxtrConf,char(169),first,last);
      | end
  Disabled : Subsystem  TreatAsAtomicUnit=on
  Merge{,1..3} (4 alike) : Merge  Inputs=3
  NoDisable : Subsystem  TreatAsAtomicUnit=on
  TimeOut : Subsystem  TreatAsAtomicUnit=on
  WhlImbRejctnDi : Outport
  PullCmpActvDi : Outport  Port=2
  InertiaCmpDecelGainDi : Outport  Port=3
  GmFctDiSts : Outport  Port=4
  wires:
  NoDisable/1(WhlImbRejctnDi) -> Merge/1
  GmFctDiSts_In/1 -> NoDisable/1(GmFctDiSts_In)
  Disabled/1(WhlImbRejctnDi) -> Merge/2
  if/1 -> TimeOut/Action
  elseif/1 -> Disabled/Action
  else/1 -> NoDisable/Action
  Merge/1 -> WhlImbRejctnDi/1
  Merge1/1 -> PullCmpActvDi/1
  Merge2/1 -> InertiaCmpDecelGainDi/1
  Merge3/1 -> GmFctDiSts/1
  TimeOut/1(WhlImbRejctnDi) -> Merge/3
  NoDisable/2(PullCmpActvDi) -> Merge1/1
  Disabled/2(PullCmpActvDi) -> Merge1/2
  TimeOut/2(PullCmpActvDi) -> Merge1/3
  NoDisable/3(InertiaCmpDecelGainDi) -> Merge2/1
  Disabled/3(InertiaCmpDecelGainDi) -> Merge2/2
  TimeOut/3(InertiaCmpDecelGainDi) -> Merge2/3
  NoDisable/4(GmFctDiSts_Out) -> Merge3/1
  Disabled/4(GmFctDiSts_Out) -> Merge3/2
  TimeOut/4(GmFctDiSts_Out) -> Merge3/3

== system CF025A_GmFctDiArbn/GmFctDiArbn/GmFctDiArbnPer1/LoaSt_doesnt_equal_SwBasdMtgtn/Copyright1 ==

== system CF025A_GmFctDiArbn/GmFctDiArbn/GmFctDiArbnPer1/LoaSt_doesnt_equal_SwBasdMtgtn/FcnDi_ElpdTi ==
  FcnDi : Inport
  FcnDiStrtTi : Inport  Port=2
  Copyright1 : Subsystem  Description=|  mask(Copyright Information){none=on}
      | Copyright info block.                                               
      |                                                                     
      | Place copyright information at the top of every subsystem in design.
      mask prompts: none "No parameters"
      mask help: Place copyright information at the top of every subsystem in design.
      mask Display:
      | NxtrConf = 'Nexteer Confidential';
      | 
      | sys = bdroot; %handle for the current model ("system")
      | first = get_param(sys,'Created');
      | if(isempty(first))
      |     first = datestr(now,'yyyy');
      | else
      |     first = first(end-3:end);  %year is last four digits
      | end
      | 
      | last = get_param(sys,'LastModifiedDate');
      | if isempty(last)
      |     last = datestr(now,'yyyy');
      | else
      |     last = last(end-3:end);
      | end
      | 
      | if strcmp(first,last)
      |     fprintf('%s\nCopyright  %s Nexteer',NxtrConf,first);
      | else
      |     fprintf('%s\n%s%s-%s Nexteer',NxtrConf,char(169),first,last);
      | end
  ElpdTi_TiPassd : Subsystem  TreatAsAtomicUnit=on
  ElpdTi_Zero : Subsystem  TreatAsAtomicUnit=on
  If : If  IfExpression=u1
  Merge : Merge
  ElpdTi : Outport
  wires:
  If/1 -> ElpdTi_TiPassd/Action
  FcnDi/1 -> If/1
  Merge/1 -> ElpdTi/1
  ElpdTi_Zero/1(ElpdTi) -> Merge/2
  If/2 -> ElpdTi_Zero/Action
  ElpdTi_TiPassd/1(ElpdTi) -> Merge/1
  FcnDiStrtTi/1 -> ElpdTi_TiPassd/1(FcnDiStrtTi)

== system CF025A_GmFctDiArbn/GmFctDiArbn/GmFctDiReq/GetRefTmr100MicroSec32bit/CopyRight2 ==

== system CF025A_GmFctDiArbn/GmFctDiArbn/GmFctDiArbnPer1/LoaSt_doesnt_equal_SwBasdMtgtn/CheckEotPosInRange/Copyright1 ==

== system CF025A_GmFctDiArbn/GmFctDiArbn/GmFctDiArbnPer1/LoaSt_doesnt_equal_SwBasdMtgtn/CheckEotPosInRange/InProc ==
  note: Need timers for being at the EOT
  HwAgFinal : Inport
  CwEot : Inport  Port=2
  CcwEot : Inport  Port=3
  Action Port : ActionPort  ActionType=then
  Constant7 : Constant  Value=ZEROHWAG_HWDEG_F32
  Copyright1 : Subsystem  Description=|  mask(Copyright Information){none=on}
      | Copyright info block.                                               
      |                                                                     
      | Place copyright information at the top of every subsystem in design.
      mask prompts: none "No parameters"
      mask help: Place copyright information at the top of every subsystem in design.
      mask Display:
      | NxtrConf = 'Nexteer Confidential';
      | 
      | sys = bdroot; %handle for the current model ("system")
      | first = get_param(sys,'Created');
      | if(isempty(first))
      |     first = datestr(now,'yyyy');
      | else
      |     first = first(end-3:end);  %year is last four digits
      | end
      | 
      | last = get_param(sys,'LastModifiedDate');
      | if isempty(last)
      |     last = datestr(now,'yyyy');
      | else
      |     last = last(end-3:end);
      | end
      | 
      | if strcmp(first,last)
      |     fprintf('%s\nCopyright  %s Nexteer',NxtrConf,first);
      | else
      |     fprintf('%s\n%s%s-%s Nexteer',NxtrConf,char(169),first,last);
      | end
  Enumerated Constant : simulink/Sources/Enumerated Constant  OutDataTypeStr=Enum: GmFctDiArbnSts1  Value=GmFctDiArbnSts1.GMFCTDIARBNSTS_INPROC  SampleTime=inf
  If : If  IfExpression=u1
  InRangeCcwDirection : Subsystem  TreatAsAtomicUnit=on
  InRangeCwDirection : Subsystem  TreatAsAtomicUnit=on
  SteeringDirection : RelationalOperator  Operator=>  OutDataTypeStr=boolean
  GmFctDiSts_InProc : Outport
  wires:
  If/2 -> InRangeCcwDirection/Action
  CcwEot/1 -> InRangeCcwDirection/1(CcwEot)
  SteeringDirection/1 -> If/1  "SteeringDirection"
  If/1 -> InRangeCwDirection/Action
  CwEot/1 -> InRangeCwDirection/1(CwEot)
  Constant7/1 -> SteeringDirection/2
  HwAgFinal/1 -> InRangeCcwDirection/2(HwAgFinal), InRangeCwDirection/2(HwAgFinal), SteeringDirection/1
  Enumerated Constant/1 -> GmFctDiSts_InProc/1

== system CF025A_GmFctDiArbn/GmFctDiArbn/GmFctDiArbnPer1/LoaSt_doesnt_equal_SwBasdMtgtn/CheckEotPosInRange/Wait ==
  Action Port : ActionPort  ActionType=else
  Constant3 : Constant  Value=false
  Constant4 : Constant  Value=false
  Copyright1 : Subsystem  Description=|  mask(Copyright Information){none=on}
      | Copyright info block.                                               
      |                                                                     
      | Place copyright information at the top of every subsystem in design.
      mask prompts: none "No parameters"
      mask help: Place copyright information at the top of every subsystem in design.
      mask Display:
      | NxtrConf = 'Nexteer Confidential';
      | 
      | sys = bdroot; %handle for the current model ("system")
      | first = get_param(sys,'Created');
      | if(isempty(first))
      |     first = datestr(now,'yyyy');
      | else
      |     first = first(end-3:end);  %year is last four digits
      | end
      | 
      | last = get_param(sys,'LastModifiedDate');
      | if isempty(last)
      |     last = datestr(now,'yyyy');
      | else
      |     last = last(end-3:end);
      | end
      | 
      | if strcmp(first,last)
      |     fprintf('%s\nCopyright  %s Nexteer',NxtrConf,first);
      | else
      |     fprintf('%s\n%s%s-%s Nexteer',NxtrConf,char(169),first,last);
      | end
  Data Store Write3 : DataStoreWrite  DataStoreName=CcwEotEnad
  Data Store Write4 : DataStoreWrite  DataStoreName=CwEotEnad
  Enumerated Constant : simulink/Sources/Enumerated Constant  OutDataTypeStr=Enum: GmFctDiArbnSts1  Value=GmFctDiArbnSts1.GMFCTDIARBNSTS_WAIT  SampleTime=inf
  GmFctDiSts_Wait : Outport
  wires:
  Constant3/1 -> Data Store Write3/1
  Constant4/1 -> Data Store Write4/1
  Enumerated Constant/1 -> GmFctDiSts_Wait/1

== system CF025A_GmFctDiArbn/GmFctDiArbn/GmFctDiArbnPer1/LoaSt_doesnt_equal_SwBasdMtgtn/CheckHwTqZeroAndHwAgZero/Copyright1 ==

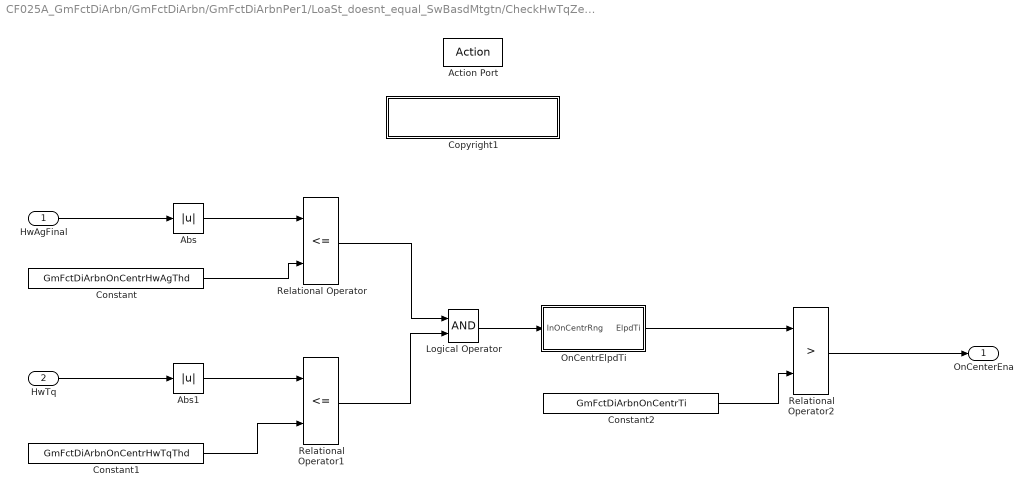
== system CF025A_GmFctDiArbn/GmFctDiArbn/GmFctDiArbnPer1/LoaSt_doesnt_equal_SwBasdMtgtn/CheckHwTqZeroAndHwAgZero/IfBothEotElpdTimeMet ==
  HwAgFinal : Inport
  HwTq : Inport  Port=2
  Action Port : ActionPort  ActionType=then
  Abs : Abs
  Abs1 : Abs
  Constant : Constant  Value=GmFctDiArbnOnCentrHwAgThd
  Constant1 : Constant  Value=GmFctDiArbnOnCentrHwTqThd
  Constant2 : Constant  Value=GmFctDiArbnOnCentrTi
  Copyright1 : Subsystem  Description=|  mask(Copyright Information){none=on}
      | Copyright info block.                                               
      |                                                                     
      | Place copyright information at the top of every subsystem in design.
      mask prompts: none "No parameters"
      mask help: Place copyright information at the top of every subsystem in design.
      mask Display:
      | NxtrConf = 'Nexteer Confidential';
      | 
      | sys = bdroot; %handle for the current model ("system")
      | first = get_param(sys,'Created');
      | if(isempty(first))
      |     first = datestr(now,'yyyy');
      | else
      |     first = first(end-3:end);  %year is last four digits
      | end
      | 
      | last = get_param(sys,'LastModifiedDate');
      | if isempty(last)
      |     last = datestr(now,'yyyy');
      | else
      |     last = last(end-3:end);
      | end
      | 
      | if strcmp(first,last)
      |     fprintf('%s\nCopyright  %s Nexteer',NxtrConf,first);
      | else
      |     fprintf('%s\n%s%s-%s Nexteer',NxtrConf,char(169),first,last);
      | end
  Logical Operator : Logic  AllPortsSameDT=off  OutDataTypeStr=boolean
  OnCentrElpdTi : Subsystem
  Relational Operator : RelationalOperator  Operator=<=  OutDataTypeStr=boolean
  Relational Operator1 : RelationalOperator  Operator=<=  OutDataTypeStr=boolean
  Relational Operator2 : RelationalOperator  Operator=>  OutDataTypeStr=boolean
  OnCenterEna : Outport
  wires:
  HwAgFinal/1 -> Abs/1
  Abs/1 -> Relational Operator/1
  Constant/1 -> Relational Operator/2
  HwTq/1 -> Abs1/1
  Abs1/1 -> Relational Operator1/1
  Constant1/1 -> Relational Operator1/2
  Relational Operator/1 -> Logical Operator/1
  Relational Operator1/1 -> Logical Operator/2
  Logical Operator/1 -> OnCentrElpdTi/1(InOnCentrRng)
  OnCentrElpdTi/1(ElpdTi) -> Relational Operator2/1
  Constant2/1 -> Relational Operator2/2
  Relational Operator2/1 -> OnCenterEna/1

== system CF025A_GmFctDiArbn/GmFctDiArbn/GmFctDiArbnPer1/LoaSt_doesnt_equal_SwBasdMtgtn/ComponentDisable/Copyright1 ==

== system CF025A_GmFctDiArbn/GmFctDiArbn/GmFctDiArbnPer1/LoaSt_doesnt_equal_SwBasdMtgtn/ComponentDisable/Disabled ==
  note: Latch stays in effect for the remainder of the key cycle
  Action Port : ActionPort  ActionType=elseif
  Constant{,1..3} (4 alike) : Constant  Value=true
  Copyright1 : Subsystem  Description=|  mask(Copyright Information){none=on}
      | Copyright info block.                                               
      |                                                                     
      | Place copyright information at the top of every subsystem in design.
      mask prompts: none "No parameters"
      mask help: Place copyright information at the top of every subsystem in design.
      mask Display:
      | NxtrConf = 'Nexteer Confidential';
      | 
      | sys = bdroot; %handle for the current model ("system")
      | first = get_param(sys,'Created');
      | if(isempty(first))
      |     first = datestr(now,'yyyy');
      | else
      |     first = first(end-3:end);  %year is last four digits
      | end
      | 
      | last = get_param(sys,'LastModifiedDate');
      | if isempty(last)
      |     last = datestr(now,'yyyy');
      | else
      |     last = last(end-3:end);
      | end
      | 
      | if strcmp(first,last)
      |     fprintf('%s\nCopyright  %s Nexteer',NxtrConf,first);
      | else
      |     fprintf('%s\n%s%s-%s Nexteer',NxtrConf,char(169),first,last);
      | end
  Data Store Write1 : DataStoreWrite  DataStoreName=FctDiLtch
  Enumerated Constant : simulink/Sources/Enumerated Constant  OutDataTypeStr=Enum: GmFctDiArbnSts1  Value=GmFctDiArbnSts1.GMFCTDIARBNSTS_PASSD  SampleTime=inf
  WhlImbRejctnDi : Outport
  PullCmpActvDi : Outport  Port=2
  InertiaCmpDecelGainDi : Outport  Port=3
  GmFctDiSts_Out : Outport  Port=4
  wires:
  Constant/1 -> Data Store Write1/1
  Constant1/1 -> WhlImbRejctnDi/1
  Constant2/1 -> PullCmpActvDi/1
  Constant3/1 -> InertiaCmpDecelGainDi/1
  Enumerated Constant/1 -> GmFctDiSts_Out/1

== system CF025A_GmFctDiArbn/GmFctDiArbn/GmFctDiArbnPer1/LoaSt_doesnt_equal_SwBasdMtgtn/ComponentDisable/NoDisable ==
  GmFctDiSts_In : Inport
  Action Port : ActionPort  ActionType=else
  Constant1 : Constant  Value=false
  Constant2 : Constant  Value=false
  Constant3 : Constant  Value=false
  Copyright1 : Subsystem  Description=|  mask(Copyright Information){none=on}
      | Copyright info block.                                               
      |                                                                     
      | Place copyright information at the top of every subsystem in design.
      mask prompts: none "No parameters"
      mask help: Place copyright information at the top of every subsystem in design.
      mask Display:
      | NxtrConf = 'Nexteer Confidential';
      | 
      | sys = bdroot; %handle for the current model ("system")
      | first = get_param(sys,'Created');
      | if(isempty(first))
      |     first = datestr(now,'yyyy');
      | else
      |     first = first(end-3:end);  %year is last four digits
      | end
      | 
      | last = get_param(sys,'LastModifiedDate');
      | if isempty(last)
      |     last = datestr(now,'yyyy');
      | else
      |     last = last(end-3:end);
      | end
      | 
      | if strcmp(first,last)
      |     fprintf('%s\nCopyright  %s Nexteer',NxtrConf,first);
      | else
      |     fprintf('%s\n%s%s-%s Nexteer',NxtrConf,char(169),first,last);
      | end
  WhlImbRejctnDi : Outport
  PullCmpActvDi : Outport  Port=2
  InertiaCmpDecelGainDi : Outport  Port=3
  GmFctDiSts_Out : Outport  Port=4
  wires:
  Constant3/1 -> InertiaCmpDecelGainDi/1
  Constant2/1 -> PullCmpActvDi/1
  Constant1/1 -> WhlImbRejctnDi/1
  GmFctDiSts_In/1 -> GmFctDiSts_Out/1
